simulink model "SimulationFromTVCPaper"  (R2022b)
settings: Solver=VariableStepAuto  StartTime=0.0  StopTime=10.0  RelTol=1e-3
PreLoadFcn:
  | ParametersFromTVCpaper
values from neighbouring files (symbols this model uses):
  CN = CN_INTERFERENCE + CN_BODY + CN_NOSE + CN_FINS    [ParametersFromTVCpaper.m]
  cross_sectional_area = pi*max_diameter^2 /4    (= 0.0452389342117)    [ParametersFromTVCpaper.m]
  g = [0,0,-9.81]    [InitParams.m]    (also in ParametersFromTVCpaper.m = 9.81)
  J_vec = [0.034, 6.3, 6.3]    [ParametersFromTVCpaper.m]
  kinematic_viscosity = 1.495*10^-5    (= 1.495e-05)    [ParametersFromTVCpaper.m]
  rocket_length = 3.57    [ParametersFromTVCpaper.m]
  Thrust = 50    [ParametersFromTVCpaper.m]
  total_mass = 82.9    [ParametersFromTVCpaper.m]
libraries: matrix_library x4, aerolibatmos2 x1
settings Model: Creator=nikil  LastModifiedBy=nikil

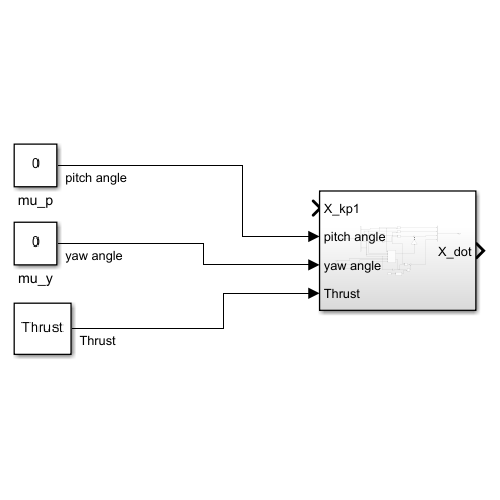
[thumbnail: Simulink's stored preview of the top-level diagram]
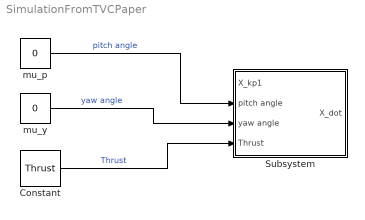
== system SimulationFromTVCPaper ==
  Constant : Constant  Value=Thrust
  Subsystem : Subsystem
  mu_p : Constant  Value=0
  mu_y : Constant  Value=0
  wires:
  mu_p/1 -> Subsystem/2(pitch angle)  "pitch angle"
  mu_y/1 -> Subsystem/3(yaw angle)  "yaw angle"
  Constant/1 -> Subsystem/4(Thrust)  "Thrust"

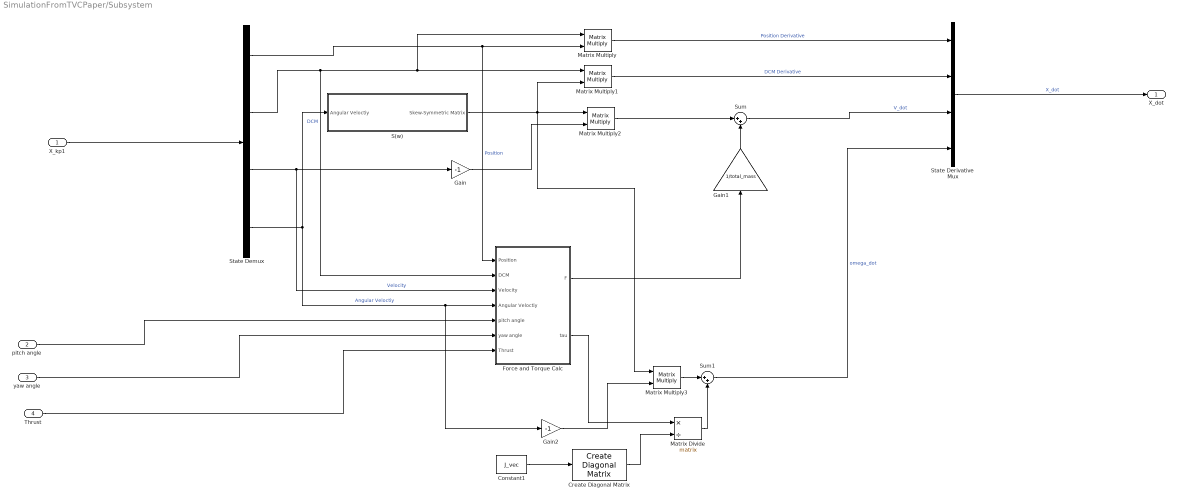
== system SimulationFromTVCPaper/Subsystem ==
  X_kp1 : Inport
  pitch angle : Inport  Port=2
  yaw angle : Inport  Port=3
  Thrust : Inport  Port=4
  Constant1 : Constant  Value=J_vec
  Create Diagonal Matrix : matrix_library/Create Diagonal Matrix
      settings: LibrarySourceBlock=|
      | simulink/Matrix
      | Operations/Create Diagonal
      | Matrix
  Force and Torque Calc : Subsystem
  Gain : Gain  Gain=-1
  Gain1 : Gain  Gain=1/total_mass
  Gain2 : Gain  Gain=-1
  Matrix Divide : Product  Inputs=*/  Multiplication=Matrix(*)
  Matrix Multiply{,1..3} (4 alike) : Product  Multiplication=Matrix(*)
  S(w) : Subsystem
  State Demux : Demux
  State Derivative Mux : Mux
  Sum : Sum  Inputs=|++
  Sum1 : Sum  Inputs=|++
  X_dot : Outport
  wires:
  Gain1/1 -> Sum/2
  State Demux/3 -> Force and Torque Calc/3(Velocity), Gain/1  "Velocity"
  S(w)/1(Skew-Symmetric Matrix) -> Matrix Multiply3/1, Matrix Multiply1/2, Matrix Multiply2/1
  Matrix Multiply/1 -> State Derivative Mux/1  "Position Derivative"
  Gain/1 -> Matrix Multiply2/2
  State Demux/2 -> Matrix Multiply1/1, Matrix Multiply/1, Force and Torque Calc/2(DCM)  "DCM"
  Matrix Multiply3/1 -> Sum1/1
  State Derivative Mux/1 -> X_dot/1  "X_dot"
  State Demux/1 -> Force and Torque Calc/1(Position), Matrix Multiply/2  "Position"
  Matrix Multiply1/1 -> State Derivative Mux/2  "DCM Derivative"
  Matrix Multiply2/1 -> Sum/1
  State Demux/4 -> Gain2/1, Force and Torque Calc/4(Angular Veloctiy), S(w)/1(Angular Veloctiy)  "Angular Veloctiy"
  Create Diagonal Matrix/1 -> Matrix Divide/2
  Force and Torque Calc/2(tau) -> Matrix Divide/1
  Sum1/1 -> State Derivative Mux/4  "omega_dot"
  yaw angle/1 -> Force and Torque Calc/6(yaw angle)
  Matrix Divide/1 -> Sum1/2
  Constant1/1 -> Create Diagonal Matrix/1
  Sum/1 -> State Derivative Mux/3  "V_dot"
  Gain2/1 -> Matrix Multiply3/2
  Force and Torque Calc/1(F) -> Gain1/1
  Thrust/1 -> Force and Torque Calc/7(Thrust)
  pitch angle/1 -> Force and Torque Calc/5(pitch angle)
  X_kp1/1 -> State Demux/1

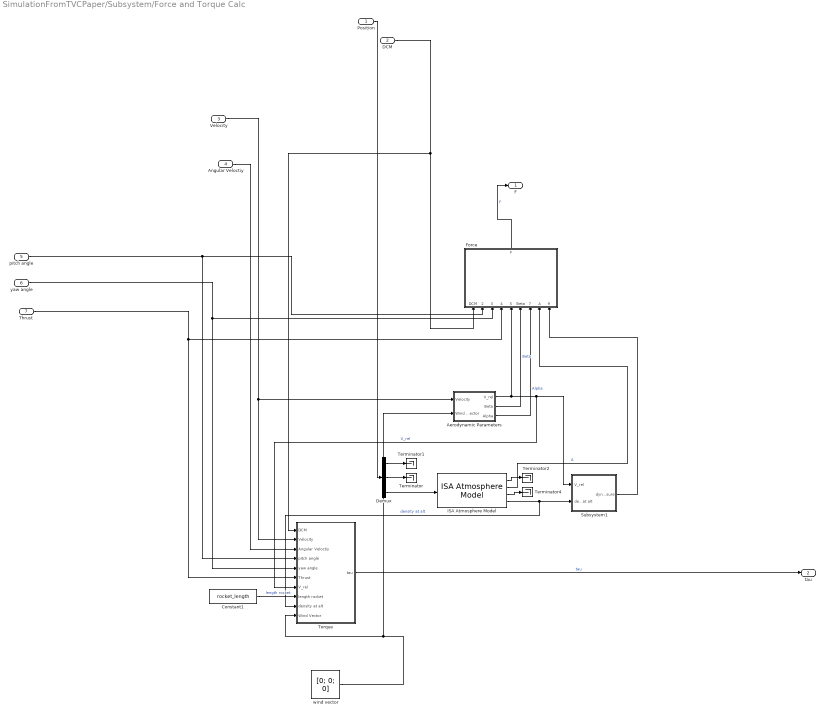
== system SimulationFromTVCPaper/Subsystem/Force and Torque Calc ==
  Position : Inport
  DCM : Inport  Port=2
  Velocity : Inport  Port=3
  Angular Veloctiy : Inport  Port=4
  pitch angle : Inport  Port=5
  yaw angle : Inport  Port=6
  Thrust : Inport  Port=7
  Aerodynamic Parameters : Subsystem
  Constant1 : Constant  Value=rocket_length
  Demux : Demux  Outputs=3
  Force : Subsystem
  ISA Atmosphere Model : aerolibatmos2/ISA Atmosphere Model  custom=off  g=9.80665  gamma=1.4  R=287.0531  L=0.0065  h_trop=11000  h_strat=20000  rho0=1.225  P0=101325  T0=288.15  h0=0
  Subsystem1 : Subsystem
  Terminator{,1..2,4} (4 alike) : Terminator
  Torque : Subsystem
  wind vector : Constant  Value=[0; 0; 0]  VectorParams1D=off
  F : Outport
  tau : Outport  Port=2
  wires:
  Angular Veloctiy/1 -> Torque/3(Angular Veloctiy)
  yaw angle/1 -> Torque/5(yaw angle), Force/3(yaw angle)
  pitch angle/1 -> Torque/4(pitch angle), Force/2(pitch angle)
  wind vector/1 -> Torque/10(Wind Vector), Aerodynamic Parameters/2(Wind Vector)
  ISA Atmosphere Model/3 -> Terminator4/1
  Aerodynamic Parameters/1(V_rel) -> Subsystem1/1(V_rel), Torque/7(V_rel), Force/5(V_rel)  "V_rel"
  ISA Atmosphere Model/1 -> Terminator2/1
  Constant1/1 -> Torque/8(length rocket)  "length rocket"
  Demux/2 -> Terminator/1
  Demux/1 -> Terminator1/1
  Demux/3 -> ISA Atmosphere Model/1
  Thrust/1 -> Force/4(Thrust), Torque/6(Thrust)
  ISA Atmosphere Model/4 -> Torque/9(density at alt), Subsystem1/2(density at alt)  "density at alt"
  Force/1(F) -> F/1  "F"
  Aerodynamic Parameters/2(Beta) -> Force/6(Beta)  "Beta"
  Aerodynamic Parameters/3(Alpha) -> Force/7(Alpha)  "Alpha"
  Subsystem1/1(dynamicPressure) -> Force/9(dynamic Pressure)
  ISA Atmosphere Model/2 -> Force/8(A)  "A"
  DCM/1 -> Torque/1(DCM), Force/1(DCM)
  Position/1 -> Demux/1
  Velocity/1 -> Aerodynamic Parameters/1(Velocity), Torque/2(Velocity)
  Torque/1(tau) -> tau/1  "tau"

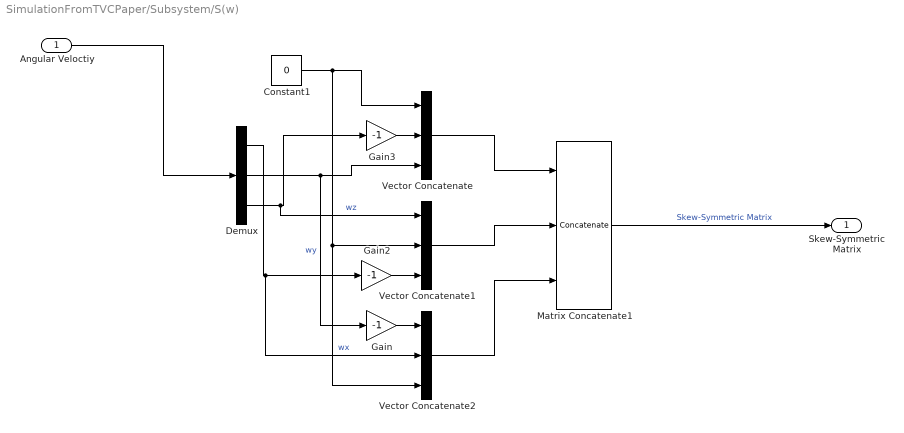
== system SimulationFromTVCPaper/Subsystem/S(w) ==
  Angular Veloctiy : Inport
  Constant1 : Constant  Value=0
  Demux : Demux  Outputs=3
  Gain : Gain  Gain=-1
  Gain2 : Gain  Gain=-1
  Gain3 : Gain  Gain=-1
  Matrix Concatenate1 : Concatenate  NumInputs=3  ConcatenateDimension=2
  Vector Concatenate : Concatenate  NumInputs=3
  Vector Concatenate1 : Concatenate  NumInputs=3
  Vector Concatenate2 : Concatenate  NumInputs=3
  Skew-Symmetric Matrix : Outport
  wires:
  Vector Concatenate2/1 -> Matrix Concatenate1/3
  Vector Concatenate/1 -> Matrix Concatenate1/1
  Gain2/1 -> Vector Concatenate1/3
  Constant1/1 -> Vector Concatenate2/3, Vector Concatenate1/2, Vector Concatenate/1
  Gain3/1 -> Vector Concatenate/2
  Demux/1 -> Vector Concatenate2/2, Gain2/1  "wx"
  Demux/3 -> Vector Concatenate1/1, Gain3/1  "wz"
  Demux/2 -> Vector Concatenate/3, Gain/1  "wy"
  Vector Concatenate1/1 -> Matrix Concatenate1/2
  Gain/1 -> Vector Concatenate2/1
  Matrix Concatenate1/1 -> Skew-Symmetric Matrix/1  "Skew-Symmetric Matrix"
  Angular Veloctiy/1 -> Demux/1

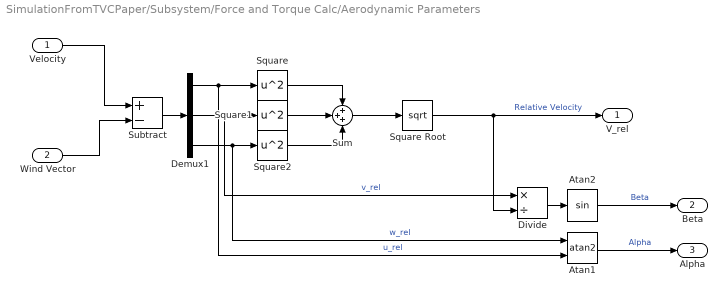
== system SimulationFromTVCPaper/Subsystem/Force and Torque Calc/Aerodynamic Parameters ==
  Velocity : Inport
  Wind Vector : Inport  Port=2
  Atan1 : Trigonometry  Operator=atan2
  Atan2 : Trigonometry
  Demux1 : Demux  Outputs=3
  Divide : Product  Inputs=*/
  Square : Math  Operator=square
  Square Root : Sqrt
  Square1 : Math  Operator=square
  Square2 : Math  Operator=square
  Subtract : Sum  Inputs=+-
  Sum : Sum  Inputs=+++
  V_rel : Outport
  Beta : Outport  Port=2
  Alpha : Outport  Port=3
  wires:
  Demux1/1 -> Atan1/2, Square/1  "u_rel"
  Sum/1 -> Square Root/1
  Square/1 -> Sum/1
  Demux1/3 -> Atan1/1, Square2/1  "w_rel"
  Square2/1 -> Sum/3
  Square1/1 -> Sum/2
  Demux1/2 -> Divide/1, Square1/1  "v_rel"
  Square Root/1 -> Divide/2, V_rel/1  "Relative Velocity"
  Velocity/1 -> Subtract/1
  Wind Vector/1 -> Subtract/2
  Subtract/1 -> Demux1/1
  Atan2/1 -> Beta/1  "Beta"
  Atan1/1 -> Alpha/1  "Alpha"
  Divide/1 -> Atan2/1

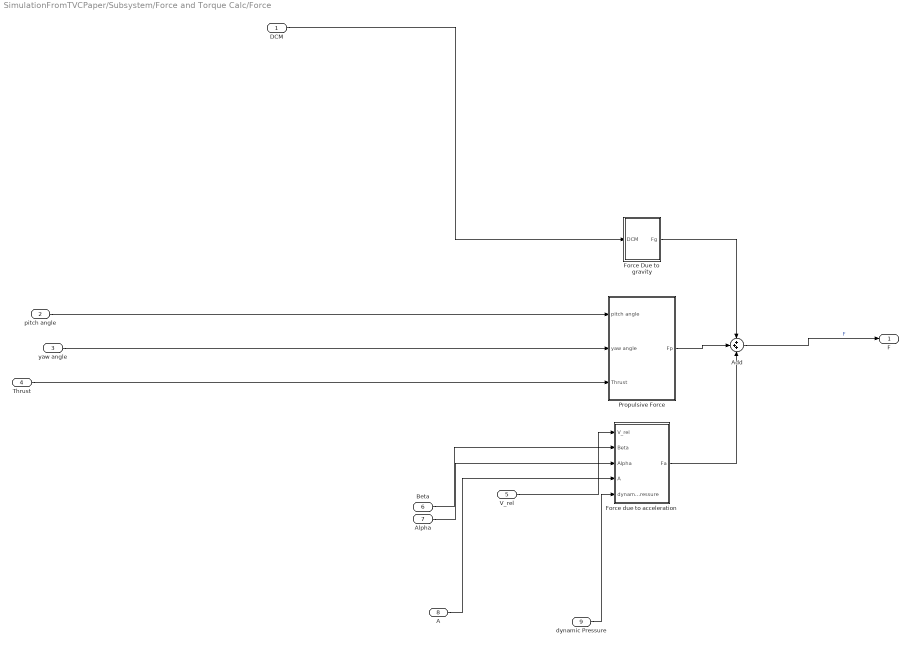
== system SimulationFromTVCPaper/Subsystem/Force and Torque Calc/Force ==
  DCM : Inport
  pitch angle : Inport  Port=2
  yaw angle : Inport  Port=3
  Thrust : Inport  Port=4
  V_rel : Inport  Port=5
  Beta : Inport  Port=6
  Alpha : Inport  Port=7
  A : Inport  Port=8
  dynamic Pressure : Inport  Port=9
  Add : Sum  Inputs=+++
  Force Due to gravity : Subsystem
  Force due to acceleration : Subsystem
  Propulsive Force : Subsystem
  F : Outport
  wires:
  DCM/1 -> Force Due to gravity/1(DCM)
  Propulsive Force/1(Fp) -> Add/2
  Force Due to gravity/1(Fg) -> Add/1
  A/1 -> Force due to acceleration/4(A)
  Thrust/1 -> Propulsive Force/3(Thrust)
  Force due to acceleration/1(Fa) -> Add/3
  V_rel/1 -> Force due to acceleration/1(V_rel)
  Alpha/1 -> Force due to acceleration/3(Alpha)
  pitch angle/1 -> Propulsive Force/1(pitch angle)
  Beta/1 -> Force due to acceleration/2(Beta)
  yaw angle/1 -> Propulsive Force/2(yaw angle)
  dynamic Pressure/1 -> Force due to acceleration/5(dynamic Pressure)
  Add/1 -> F/1  "F"

== system SimulationFromTVCPaper/Subsystem/Force and Torque Calc/Subsystem1 ==
  V_rel : Inport
  density at alt : Inport  Port=2
  Constant3 : Constant  Value=0.5
  Product : Product  Inputs=3
  Square3 : Math  Operator=square
  dynamicPressure : Outport
  wires:
  Constant3/1 -> Product/1
  Square3/1 -> Product/2
  density at alt/1 -> Product/3
  V_rel/1 -> Square3/1
  Product/1 -> dynamicPressure/1  "dynamicPressure"

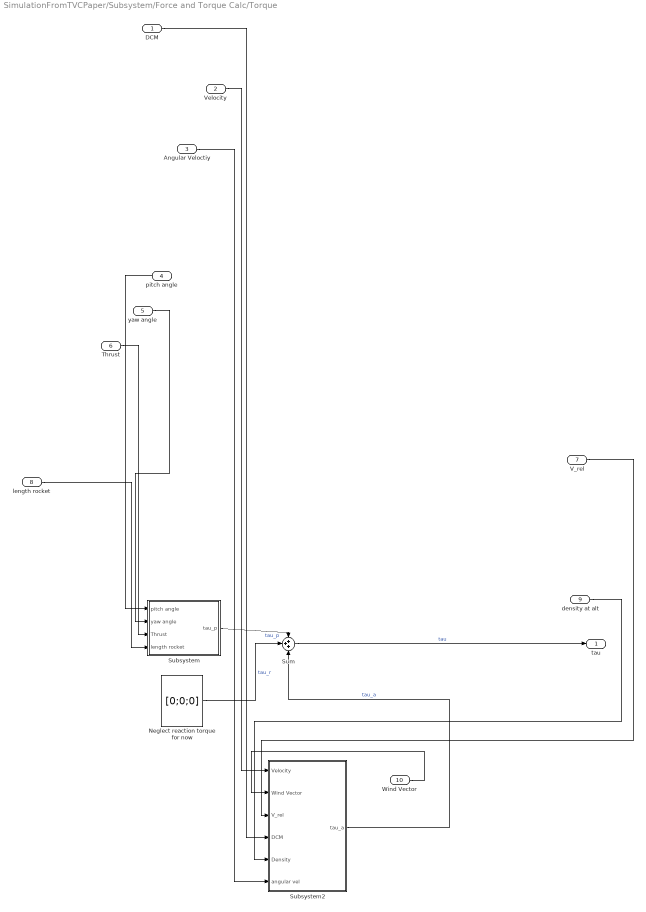
== system SimulationFromTVCPaper/Subsystem/Force and Torque Calc/Torque ==
  DCM : Inport
  Velocity : Inport  Port=2
  Angular Veloctiy : Inport  Port=3
  pitch angle : Inport  Port=4
  yaw angle : Inport  Port=5
  Thrust : Inport  Port=6
  V_rel : Inport  Port=7
  length rocket : Inport  Port=8
  density at alt : Inport  Port=9
  Wind Vector : Inport  Port=10
  Neglect reaction torque for now : Constant  Value=[0;0;0]  VectorParams1D=off
  Subsystem : Subsystem
  Subsystem2 : Subsystem
  Sum : Sum  Inputs=+++
  tau : Outport
  wires:
  yaw angle/1 -> Subsystem/2(yaw angle)
  Velocity/1 -> Subsystem2/1(Velocity)
  Sum/1 -> tau/1  "tau"
  Angular Veloctiy/1 -> Subsystem2/6(angular vel)
  density at alt/1 -> Subsystem2/5(Density)
  pitch angle/1 -> Subsystem/1(pitch angle)
  Thrust/1 -> Subsystem/3(Thrust)
  Subsystem2/1(tau_a) -> Sum/3  "tau_a"
  Neglect reaction torque for now/1 -> Sum/2  "tau_r"
  Subsystem/1(tau_p) -> Sum/1  "tau_p"
  length rocket/1 -> Subsystem/4(length rocket)
  V_rel/1 -> Subsystem2/3(V_rel)
  DCM/1 -> Subsystem2/4(DCM)
  Wind Vector/1 -> Subsystem2/2(Wind Vector)

== system SimulationFromTVCPaper/Subsystem/Force and Torque Calc/Force/Force Due to gravity ==
  DCM : Inport
  Gravity Vector : Constant  Value=[-g;0;0]  VectorParams1D=off
  Matrix Multiply3 : Product  Multiplication=Matrix(*)
  Transpose : Math  Operator=transpose
  Fg : Outport
  wires:
  Gravity Vector/1 -> Matrix Multiply3/2
  Transpose/1 -> Matrix Multiply3/1
  Matrix Multiply3/1 -> Fg/1  "Fg"
  DCM/1 -> Transpose/1

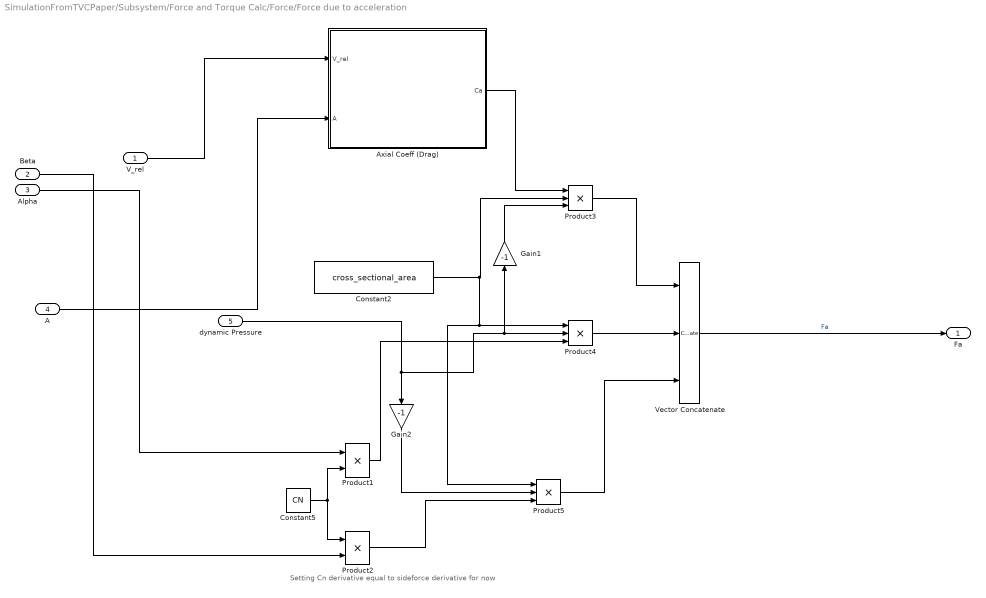
== system SimulationFromTVCPaper/Subsystem/Force and Torque Calc/Force/Force due to acceleration ==
  note: Setting Cn derivative equal to sideforce derivative for now
  V_rel : Inport
  Beta : Inport  Port=2
  Alpha : Inport  Port=3
  A : Inport  Port=4
  dynamic Pressure : Inport  Port=5
  Axial Coeff (Drag) : Subsystem
  Constant2 : Constant  Value=cross_sectional_area
  Constant5 : Constant  Value=CN
  Gain1 : Gain  Gain=-1
  Gain2 : Gain  Gain=-1
  Product1 : Product
  Product2 : Product
  Product3 : Product  Inputs=3
  Product4 : Product  Inputs=3
  Product5 : Product  Inputs=3
  Vector Concatenate : Concatenate  NumInputs=3
  Fa : Outport
  wires:
  Gain2/1 -> Product5/2
  dynamic Pressure/1 -> Gain2/1, Product4/2, Gain1/1
  Product4/1 -> Vector Concatenate/2
  Constant2/1 -> Product5/1, Product4/1, Product3/2
  Axial Coeff (Drag)/1(Ca) -> Product3/1
  Constant5/1 -> Product1/2, Product2/1
  Product1/1 -> Product4/3
  Alpha/1 -> Product1/1
  V_rel/1 -> Axial Coeff (Drag)/1(V_rel)
  Product5/1 -> Vector Concatenate/3
  Product2/1 -> Product5/3
  Beta/1 -> Product2/2
  Product3/1 -> Vector Concatenate/1
  Gain1/1 -> Product3/3
  A/1 -> Axial Coeff (Drag)/2(A)
  Vector Concatenate/1 -> Fa/1  "Fa"

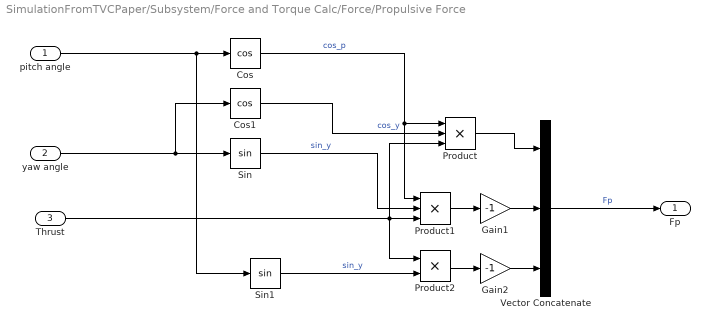
== system SimulationFromTVCPaper/Subsystem/Force and Torque Calc/Force/Propulsive Force ==
  pitch angle : Inport
  yaw angle : Inport  Port=2
  Thrust : Inport  Port=3
  Cos : Trigonometry  Operator=cos
  Cos1 : Trigonometry  Operator=cos
  Gain1 : Gain  Gain=-1
  Gain2 : Gain  Gain=-1
  Product : Product  Inputs=3
  Product1 : Product  Inputs=3
  Product2 : Product
  Sin : Trigonometry
  Sin1 : Trigonometry
  Vector Concatenate : Concatenate  NumInputs=3
  Fp : Outport
  wires:
  Cos/1 -> Product1/1, Product/1  "cos_p"
  Cos1/1 -> Product/2  "cos_y"
  Sin/1 -> Product1/2  "sin_y"
  Product/1 -> Vector Concatenate/1
  Thrust/1 -> Product2/1, Product/3, Product1/3
  Gain2/1 -> Vector Concatenate/3
  yaw angle/1 -> Cos1/1, Sin/1
  Product1/1 -> Gain1/1
  Sin1/1 -> Product2/2  "sin_y"
  Product2/1 -> Gain2/1
  pitch angle/1 -> Sin1/1, Cos/1
  Gain1/1 -> Vector Concatenate/2
  Vector Concatenate/1 -> Fp/1  "Fp"

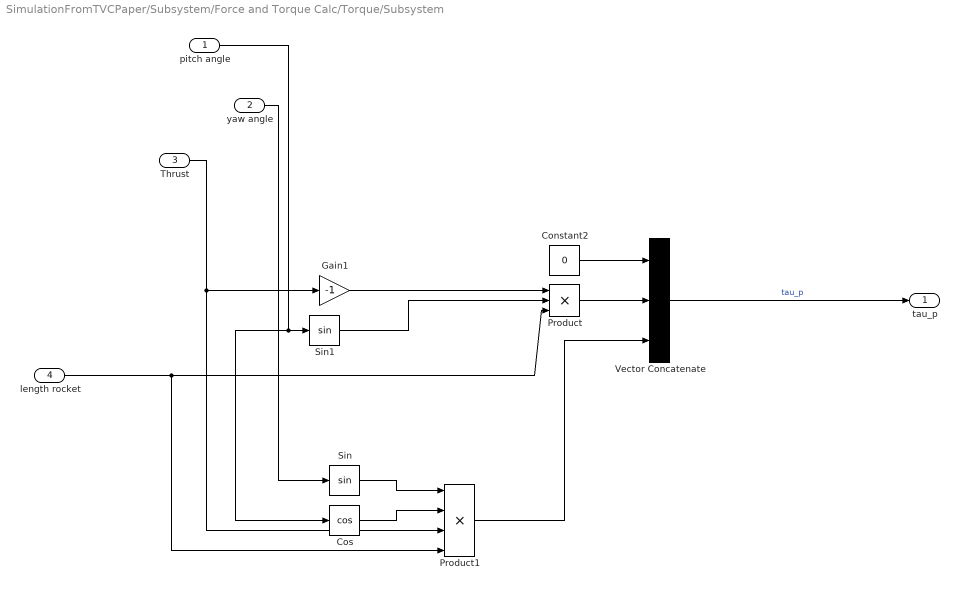
== system SimulationFromTVCPaper/Subsystem/Force and Torque Calc/Torque/Subsystem ==
  pitch angle : Inport
  yaw angle : Inport  Port=2
  Thrust : Inport  Port=3
  length rocket : Inport  Port=4
  Constant2 : Constant  Value=0
  Cos : Trigonometry  Operator=cos
  Gain1 : Gain  Gain=-1
  Product : Product  Inputs=3
  Product1 : Product  Inputs=4
  Sin : Trigonometry
  Sin1 : Trigonometry
  Vector Concatenate : Concatenate  NumInputs=3
  tau_p : Outport
  wires:
  pitch angle/1 -> Cos/1, Sin1/1
  Constant2/1 -> Vector Concatenate/1
  Sin1/1 -> Product/2
  Thrust/1 -> Product1/3, Gain1/1
  Cos/1 -> Product1/2
  Product1/1 -> Vector Concatenate/3
  Sin/1 -> Product1/1
  length rocket/1 -> Product1/4, Product/3
  yaw angle/1 -> Sin/1
  Vector Concatenate/1 -> tau_p/1  "tau_p"
  Product/1 -> Vector Concatenate/2
  Gain1/1 -> Product/1

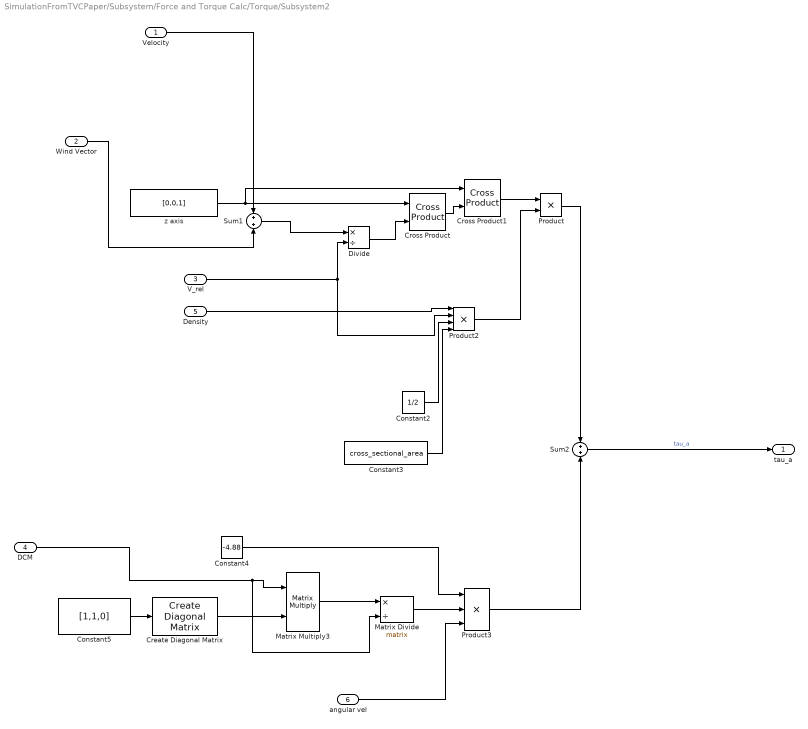
== system SimulationFromTVCPaper/Subsystem/Force and Torque Calc/Torque/Subsystem2 ==
  Velocity : Inport
  Wind Vector : Inport  Port=2
  V_rel : Inport  Port=3
  DCM : Inport  Port=4
  Density : Inport  Port=5
  angular vel : Inport  Port=6
  Constant2 : Constant  Value=1/2
  Constant3 : Constant  Value=cross_sectional_area
  Constant4 : Constant  Value=-4.88
  Constant5 : Constant  Value=[1,1,0]
  Create Diagonal Matrix : matrix_library/Create Diagonal Matrix
      settings: LibrarySourceBlock=|
      | simulink/Matrix
      | Operations/Create Diagonal
      | Matrix
  Cross Product : matrix_library/Cross Product
  Cross Product1 : matrix_library/Cross Product
  Divide : Product  Inputs=*/
  Matrix Divide : Product  Inputs=*/  Multiplication=Matrix(*)
  Matrix Multiply3 : Product  Multiplication=Matrix(*)
  Product : Product
  Product2 : Product  Inputs=4
  Product3 : Product  Inputs=3
  Sum1 : Sum
  Sum2 : Sum
  z axis : Constant  Value=[0,0,1]
  tau_a : Outport
  wires:
  Cross Product1/1 -> Product/1
  Sum2/1 -> tau_a/1  "tau_a"
  DCM/1 -> Matrix Divide/2, Matrix Multiply3/1
  Create Diagonal Matrix/1 -> Matrix Multiply3/2
  Sum1/1 -> Divide/1
  z axis/1 -> Cross Product1/1, Cross Product/1
  Product2/1 -> Product/2
  angular vel/1 -> Product3/3
  Product3/1 -> Sum2/2
  Matrix Multiply3/1 -> Matrix Divide/1
  Constant5/1 -> Create Diagonal Matrix/1
  Constant3/1 -> Product2/4
  Cross Product/1 -> Cross Product1/2
  Constant4/1 -> Product3/1
  Constant2/1 -> Product2/3
  Matrix Divide/1 -> Product3/2
  Product/1 -> Sum2/1
  Divide/1 -> Cross Product/2
  Density/1 -> Product2/1
  V_rel/1 -> Product2/2, Divide/2
  Velocity/1 -> Sum1/1
  Wind Vector/1 -> Sum1/2

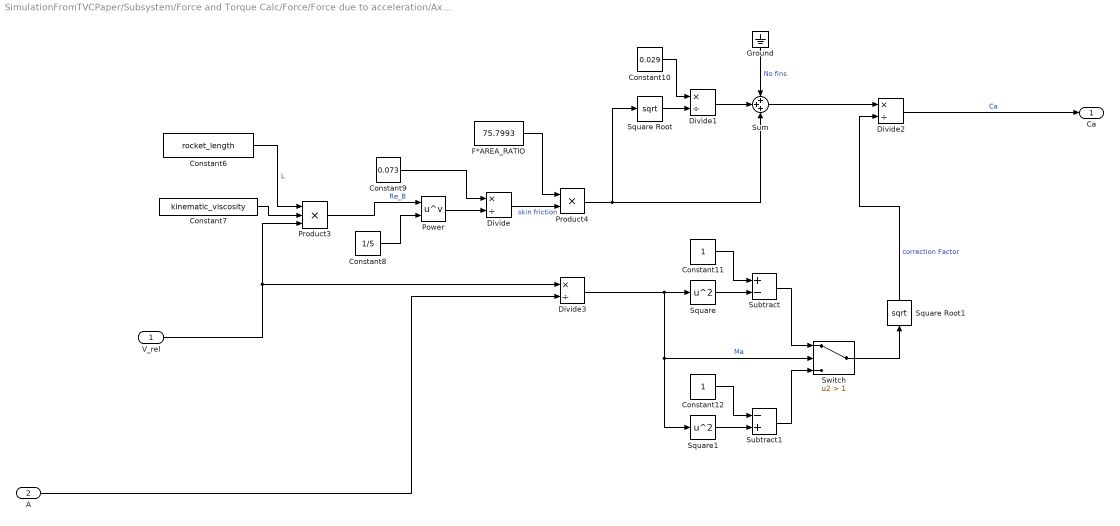
== system SimulationFromTVCPaper/Subsystem/Force and Torque Calc/Force/Force due to acceleration/Axial Coeff (Drag) ==
  V_rel : Inport
  A : Inport  Port=2
  Constant10 : Constant  Value=0.029
  Constant11 : Constant
  Constant12 : Constant
  Constant6 : Constant  Value=rocket_length
  Constant7 : Constant  Value=kinematic_viscosity
  Constant8 : Constant  Value=1/5
  Constant9 : Constant  Value=0.073
  Divide{,1..3} (4 alike) : Product  Inputs=*/
  F*AREA_RATIO : Constant  Value=75.7993
  Ground : Ground
  Power : Math  Operator=pow
  Product3 : Product  Inputs=3
  Product4 : Product
  Square : Math  Operator=square
  Square Root : Sqrt
  Square Root1 : Sqrt
  Square1 : Math  Operator=square
  Subtract : Sum  Inputs=+-
  Subtract1 : Sum  Inputs=-+
  Sum : Sum  Inputs=+++
  Switch : Switch  Criteria=u2 > Threshold  Threshold=1  SaturateOnIntegerOverflow=off  InputSameDT=off
  Ca : Outport
  wires:
  Product3/1 -> Power/1  "Re_B"
  Product4/1 -> Sum/3, Square Root/1
  Constant9/1 -> Divide/1
  Square1/1 -> Subtract1/2
  Square/1 -> Subtract/2
  Constant6/1 -> Product3/1  "L"
  F*AREA_RATIO/1 -> Product4/1
  Constant8/1 -> Power/2
  V_rel/1 -> Product3/3, Divide3/1
  Subtract1/1 -> Switch/3
  Divide1/1 -> Sum/2
  Constant11/1 -> Subtract/1
  Square Root1/1 -> Divide2/2  "correction Factor"
  Subtract/1 -> Switch/1
  Square Root/1 -> Divide1/2
  Constant10/1 -> Divide1/1
  Divide3/1 -> Square/1, Square1/1, Switch/2  "Ma"
  Divide/1 -> Product4/2  "skin friction"
  Constant12/1 -> Subtract1/1
  Constant7/1 -> Product3/2
  Ground/1 -> Sum/1  "No fins"
  Power/1 -> Divide/2
  Sum/1 -> Divide2/1
  Switch/1 -> Square Root1/1
  A/1 -> Divide3/2
  Divide2/1 -> Ca/1  "Ca"
